simulink model "realTime_lowpass_filter"  (R2020a)
settings: Solver=VariableStepAuto  StartTime=0.0  StopTime=10.0  RelTol=1e-3
libraries: audiosources x1, dspfdesign x1, dspsnks4 x1
settings Model: Creator=Karan  LastModifiedBy=Karan

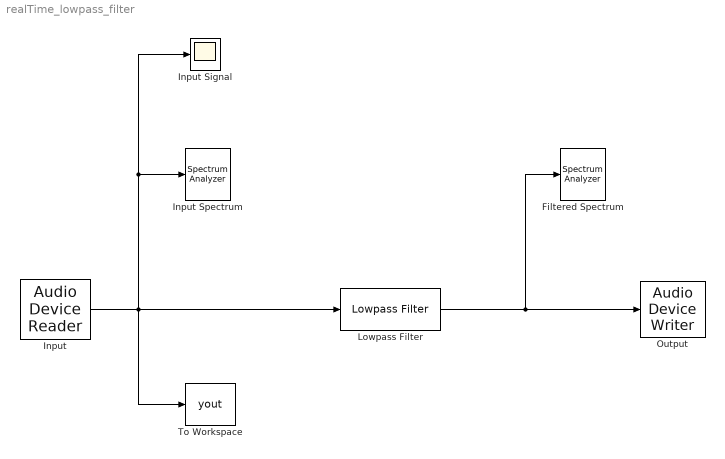
== system realTime_lowpass_filter ==
  "Filtered Spectrum " : SpectrumAnalyzer
  Input : audiosources/Audio Device Reader  Driver=DirectSound  Device=Default  SampleRate=44100  NumChannels=1  SamplesPerFrame=1024  BitDepth=16-bit integer  NumBuffers=10  DefaultInputChannelMapping=on  InputChannelMapping=1:2  OutputNumOverrunSamples=off  OutputDataType=double  DriverIdx=1  DeviceWarnFlag=''
      settings: SourceProductBaseCode=AU
  Input Signal : Scope
      settings: Tag=INPUT
  "Input Spectrum " : SpectrumAnalyzer
  Lowpass Filter : dspfdesign/Lowpass Filter  FilterType=FIR  DesignForMinimumOrder=on  FilterOrder=50  PassbandFrequency=8e3  StopbandFrequency=12e3  PassbandRipple=0.1  StopbandAttenuation=80  InheritSampleRate=off  SampleRate=44100  SimulateUsing=Interpreted execution  roundingMode=Floor  coeffsDataTypeStr=fixdt(1,16)
  Output : dspsnks4/Audio Device Writer  Driver=DirectSound  Device=Default  InheritSampleRate=on  SampleRate=44100  BitDepth=16-bit integer  BufferSize=4096  NumBuffers=10  DefaultOutputChannelMapping=on  OutputChannelMapping=1:2  OutputNumUnderrunSamples=off  DriverIdx=1  DeviceWarnFlag=''
  To Workspace : ToWorkspace  VariableName=yout  SampleTime=-1
      settings: Save2DSignal=2-D array (concatenate along first dimension)
  wires:
  Input/1 -> "Input Spectrum "/1, Input Signal/1, Lowpass Filter/1, To Workspace/1
  Lowpass Filter/1 -> "Filtered Spectrum "/1, Output/1
